simulink model "Electrical_System_2018b_obfs"  (R2019b)
settings: Solver=VariableStepAuto  StartTime=0.0  StopTime=5  RelTol=1e-3  AbsTol=1e-3  EnableMultiTasking=on
InitFcn:
  | Steady_State_Initialisation;
StopFcn:
  | %sscexplore(simlog);
  | %Logging
undefined symbols (not defined in the file): abrlhklxvp, aexgmhuedq, afmfmjnutg, afpphrjpnc, ahuxbyvruc, alarvljztt, amxnyqmnuw, aodrlwvqie, aolhmuplyq, aqpmguuqkg, auesgwirzl, aurophlnng, awamelrhru, ayfhvxflxn, azxkacuhqc, babszerikg, bawhdqanwq, bevoqecvei, bltjvqbchx, bmqsuewujl, bsmyqjfgnf, btvjbsmnve, bywgxqeadw, bziaduxaer, bzmcmdqocb, bzsvyvetat, ccsjnrbsih, cdvenygxwh, cedkrnslhx, cjheorclzs, cjrdshrtqx, ckhavyhcza, ckxewznhlz, cmrcgyiplk, conenicnws, cqkejbgjnn, csfnuwymhe, cunupkhwbh, cwzfvzuxxh, dcadmadufn, dcfponivnv, ddtrqjrhjn, dfhoxvkqas, dfrhtcwpne, dfvomcagjv, djijwylxea, dnmeqksrrm, dnzewbdkaa, dsqcykyxav, dtswwlttmm, ecumpidjtv, edegaywrct, ejjjsmnejc, eknqnehjdz, emvdetzouf, esxbqkbahr, etnkkbreiq, eunoiiiirw, ewewcuedir, fatkfxdhtc ... (+386)
libraries: fl_lib x802, ee_lib x362, fl_ps_legacy_lib x160, nesl_utility x85
(part 9 of 26)

== system Electrical_System_2018b_obfs/Redacted_1221/Redacted_7996/Redacted_1/Redacted_4377/Redacted_6082/Redacted_1335 ==
  Redacted_1591 : ee_lib/Semiconductors & Converters/Diode  ModelType=eepsypmlnm  Vf=vsdkpxkdvt V  Ron=hvipwyltcs Ohm  Goff=pncgtdpcky S  prmExp=ywnmgnebdg  I12=pijcksfllq A  V12=sokkewuwnq V  IS=lenjbmkbmu A  ec=usrydsfczj  I1=diflzejvue A  V1=ondqlqjixt V  RS=mmlszzuage Ohm  Tmeas=npymjxtxff degC  N_series=uwgycohtvj  N_parallel=vvktvyaksv  Rz=csndwjwvcs Ohm  BV=siuhniwsas V  C_param=mqmeyzacus  CJ=pspkjiflhw pF  CJ0=mkzhvuscrv pF  VJ=cxyxmemllb V  Mgrad=kwjdstgiqi  Vvec=rfkmbedwbl V  Cvec=tzcpccccyr pF  FC=tzhyramxnn  Q_param=jtaiadwcvb  iRM=teewqjimfa A  iF=dkuaowzmzk A  didt=wswqfekgti A/us  trr_factor=vgbmpjncqd  trr=qytitrwxvl ns  Qrr=jukjiwceed s*uA  TT=vfhkswzpii ns  tau=bcxefnpqla ns  T_param=knzoykoruc  IS_T2=wmrtfwgfyn A  I1_T2=wwatewxxmj A  V1_T2=vcmdipevcj V  Tmeas2=slejovgnym degC  EG_param=yrmdwgjpga  EG=obqdoxighd eV  XTI_param=hiiulsmtnp  XTI=fzvxbjgrlx  dBVdT=tcetjpxzuo V/K  Tdevice=jhymtvpuuv degC  i_specify=off  i_priority=None  i=lxkrvrufkt A  i_nominal_specify=off  i_nominal_unit=A  i_nominal_value=fptpkrapsh  v_specify=off  v_priority=None  v=hnwpggrdrb V  v_nominal_specify=off  v_nominal_unit=V  v_nominal_value=loyliznani  i_capacitor_specify=off  i_capacitor_priority=None  i_capacitor=qntetqcfew A  i_capacitor_nominal_specify=off  i_capacitor_nominal_unit=A  i_capacitor_nominal_value=bhetqfpmna  v_capacitor_specify=off  v_capacitor_priority=None  v_capacitor=qmuuchuxyz V  v_capacitor_nominal_specify=off  v_capacitor_nominal_unit=V  v_capacitor_nominal_value=vvvpkitexs  power_dissipated_specify=off  power_dissipated_priority=None  power_dissipated=kbjvtlpgfd W  power_dissipated_nominal_specify=off  power_dissipated_nominal_unit=W  power_dissipated_nominal_value=jvdnwocntn  thermal_network_parameterization=yoawbybtkl  Rth=uknyprueob K/W  Rth_Foster=quhjgsiudl K/W  thermal_mass_parameterization=atrvywscev  thermal_mass=gtmjoozywy J/K  thermal_mass_Foster=hdtqidrsds J/K  thermal_time_constant=adrtjfdoqm s  thermal_time_constant_Foster=lcosfsblai s  thermal_mass_initial_temperatures=kqftjagahg degC
      settings: SourceProductName=Simscape Electrical  InternalSimscapePortConfiguration="{\"Bottom\":[],\"Left\":[{\"id\":\"p\",\"label\":\"\",\"type\":\"foundation.electrical.electrical\"},{\"id\":\"H\",\"label\":\"H\",\"type\":\"foundation.thermal.thermal\"}],\"Right\":[{\"id\":\"n\",\"label\":\"\",\"type\":\"foundation.electrical.electrical\"}],\"Top\":[]}"
  Redacted_1669 : ee_lib/Passive/Thermal/Thermal Resistor  R=ejjjsmnejc K/W  T_specify=off  T_priority=None  T=mbytgkvqdk K  T_nominal_specify=off  T_nominal_unit=K  T_nominal_value=uvrqbhbcsu  Q_specify=off  Q_priority=None  Q=fryoumgfor W  Q_nominal_specify=off  Q_nominal_unit=W  Q_nominal_value=qudqfymccr
      settings: SourceProductName=Simscape Electrical  SourceProductBaseCode=PS  InternalSimscapePortConfiguration="{\"Bottom\":[],\"Left\":[{\"id\":\"A\",\"label\":\"A\",\"type\":\"foundation.thermal.thermal\"}],\"Right\":[{\"id\":\"B\",\"label\":\"B\",\"type\":\"foundation.thermal.thermal\"}],\"Top\":[]}"
  Redacted_4093 : fl_lib/Electrical/Electrical Elements/Switch  R_closed=bbadzxwyew Ohm  G_open=fzmtkxgwpd 1/Ohm  Threshold=dfvomcagjv  i_specify=off  i_priority=None  i=ohbeugqvip A  i_nominal_specify=off  i_nominal_unit=A  i_nominal_value=exxqjlbakz  v_specify=off  v_priority=None  v=rdiaxwucpj V  v_nominal_specify=off  v_nominal_unit=V  v_nominal_value=azkctcjsnz
      settings: SourceProductName=Simscape
  Redacted_5466 : ee_lib/Passive/Thermal/Thermal Resistor  R=wdtmondimm K/W  T_specify=off  T_priority=None  T=wrtafdzvbh K  T_nominal_specify=off  T_nominal_unit=K  T_nominal_value=fiihiabjan  Q_specify=off  Q_priority=None  Q=ypouestzei W  Q_nominal_specify=off  Q_nominal_unit=W  Q_nominal_value=mabqlhycjh
      settings: SourceProductName=Simscape Electrical  SourceProductBaseCode=PS  InternalSimscapePortConfiguration="{\"Bottom\":[],\"Left\":[{\"id\":\"A\",\"label\":\"A\",\"type\":\"foundation.thermal.thermal\"}],\"Right\":[{\"id\":\"B\",\"label\":\"B\",\"type\":\"foundation.thermal.thermal\"}],\"Top\":[]}"
  Redacted_7324 : fl_lib/Electrical/Electrical Elements/Switch  R_closed=omfvajnpfd Ohm  G_open=ipqnezpryn 1/Ohm  Threshold=mmcsavdyob  i_specify=off  i_priority=None  i=qwnjhvyruv A  i_nominal_specify=off  i_nominal_unit=A  i_nominal_value=zmauchnwye  v_specify=off  v_priority=None  v=ufnknxdamw V  v_nominal_specify=off  v_nominal_unit=V  v_nominal_value=edufhutzre
      settings: SourceProductName=Simscape
  Redacted_9050 : ee_lib/Passive/Thermal/Thermal Resistor  R=gnxjfqgycd K/W  T_specify=off  T_priority=None  T=dtswwlttmm K  T_nominal_specify=off  T_nominal_unit=K  T_nominal_value=iuxynuhpbk  Q_specify=off  Q_priority=None  Q=etqvxuddqu W  Q_nominal_specify=off  Q_nominal_unit=W  Q_nominal_value=jpdxcuslyz
      settings: SourceProductName=Simscape Electrical  SourceProductBaseCode=PS  InternalSimscapePortConfiguration="{\"Bottom\":[],\"Left\":[{\"id\":\"A\",\"label\":\"A\",\"type\":\"foundation.thermal.thermal\"}],\"Right\":[{\"id\":\"B\",\"label\":\"B\",\"type\":\"foundation.thermal.thermal\"}],\"Top\":[]}"
  Redacted_998 : ee_lib/Semiconductors & Converters/Diode  ModelType=jjfughauiv  Vf=eaqvjmxxyg V  Ron=canwxvkyyq Ohm  Goff=fylhafqfdf S  prmExp=dyvujabdmn  I12=kttaerjvea A  V12=kesibchmqe V  IS=cnmgoowrsx A  ec=wmgmtbxlpj  I1=kbcmpxrtrl A  V1=bxdgeigcbm V  RS=aqtkcecpuq Ohm  Tmeas=jagkxxxouu degC  N_series=eijeaxwsbs  N_parallel=gnezyptovg  Rz=ccfbjkqckh Ohm  BV=ibaqbmeitx V  C_param=qbielwnwyc  CJ=zriiuwgwxe pF  CJ0=dfescxdcew pF  VJ=cbwvhwuxfk V  Mgrad=imxnoqiriq  Vvec=scyvszjglj V  Cvec=fxqxkbblsd pF  FC=oefuhmbbrj  Q_param=azpytwrwfh  iRM=vffiognxml A  iF=obozmuzsag A  didt=gxjsoognzt A/us  trr_factor=ngilewgegt  trr=udeiywtgjk ns  Qrr=lseeyedphz s*uA  TT=rsgjgrebyr ns  tau=fnsxhspmvy ns  T_param=ompevgbwln  IS_T2=czoaxjmnms A  I1_T2=fomygjynsp A  V1_T2=axnvwvykbq V  Tmeas2=acusxjthih degC  EG_param=jvdcorncji  EG=cjbueeqdfy eV  XTI_param=ksyxmxcrgv  XTI=lqwkbkflhk  dBVdT=gzrvmvfdkg V/K  Tdevice=btlrowuowx degC  i_specify=off  i_priority=None  i=cbrwwtdksz A  i_nominal_specify=off  i_nominal_unit=A  i_nominal_value=tdaqsczgka  v_specify=off  v_priority=None  v=hzgsyifftd V  v_nominal_specify=off  v_nominal_unit=V  v_nominal_value=wwgtgaavtg  i_capacitor_specify=off  i_capacitor_priority=None  i_capacitor=ghdwybcfnr A  i_capacitor_nominal_specify=off  i_capacitor_nominal_unit=A  i_capacitor_nominal_value=patoccuvbb  v_capacitor_specify=off  v_capacitor_priority=None  v_capacitor=kipgljoorb V  v_capacitor_nominal_specify=off  v_capacitor_nominal_unit=V  v_capacitor_nominal_value=dyvrmzctdc  power_dissipated_specify=off  power_dissipated_priority=None  power_dissipated=ttfhebcktj W  power_dissipated_nominal_specify=off  power_dissipated_nominal_unit=W  power_dissipated_nominal_value=repcdnmkvu  thermal_network_parameterization=fmvbkiqdne  Rth=pazmfgafaa K/W  Rth_Foster=brspocefdd K/W  thermal_mass_parameterization=ykylewhfcq  thermal_mass=lrrjyxxvqd J/K  thermal_mass_Foster=vdbqyqwkrw J/K  thermal_time_constant=exusymqbix s  thermal_time_constant_Foster=asebieqyaj s  thermal_mass_initial_temperatures=hpkeovjooi degC
      settings: SourceProductName=Simscape Electrical  InternalSimscapePortConfiguration="{\"Bottom\":[],\"Left\":[{\"id\":\"p\",\"label\":\"\",\"type\":\"foundation.electrical.electrical\"},{\"id\":\"H\",\"label\":\"H\",\"type\":\"foundation.thermal.thermal\"}],\"Right\":[{\"id\":\"n\",\"label\":\"\",\"type\":\"foundation.electrical.electrical\"}],\"Top\":[]}"
  Redacted_3665 : PMIOPort  Side=Left
  Redacted_9500 : PMIOPort  Port=2  Side=Left
  Redacted_4916 : PMIOPort  Port=3  Side=Right
  Redacted_8865 : PMIOPort  Port=4  Side=Right
  Redacted_5813 : PMIOPort  Port=5  Side=Left
  Redacted_175 : PMIOPort  Port=6  Side=Right
  connections:
  Redacted_998/LConn2 -- Redacted_5466/LConn1
  Redacted_9050/RConn1 -- Redacted_5813/RConn1
  Redacted_8865/RConn1 -- Redacted_7324/RConn2
  Redacted_4093/RConn1 -- Redacted_7324/RConn1 -- Redacted_175/RConn1
  Redacted_1669/RConn1 -- Redacted_9050/LConn1 -- Redacted_5466/RConn1
  Redacted_3665/RConn1 -- Redacted_1591/RConn1
  Redacted_1591/LConn1 -- Redacted_4093/LConn1
  Redacted_4916/RConn1 -- Redacted_4093/RConn2
  Redacted_1591/LConn2 -- Redacted_1669/LConn1
  Redacted_998/RConn1 -- Redacted_7324/LConn1
  Redacted_998/LConn1 -- Redacted_9500/RConn1

== system Electrical_System_2018b_obfs/Redacted_1221/Redacted_7996/Redacted_1/Redacted_4377/Redacted_6082/Redacted_1337 ==
  Redacted_1292 : ee_lib/Passive/Thermal/Thermal Resistor  R=gfxbaoqbci K/W  T_specify=off  T_priority=None  T=rvwtgoykrz K  T_nominal_specify=off  T_nominal_unit=K  T_nominal_value=dmbpfjxefx  Q_specify=off  Q_priority=None  Q=ozjvrxmttl W  Q_nominal_specify=off  Q_nominal_unit=W  Q_nominal_value=utwlydmrkv
      settings: SourceProductName=Simscape Electrical  SourceProductBaseCode=PS  InternalSimscapePortConfiguration="{\"Bottom\":[],\"Left\":[{\"id\":\"A\",\"label\":\"A\",\"type\":\"foundation.thermal.thermal\"}],\"Right\":[{\"id\":\"B\",\"label\":\"B\",\"type\":\"foundation.thermal.thermal\"}],\"Top\":[]}"
  Redacted_2743 : fl_lib/Electrical/Electrical Elements/Switch  R_closed=fsyfpyiukg Ohm  G_open=tvcalsacmg 1/Ohm  Threshold=ttjzchmxti  i_specify=off  i_priority=None  i=alduyvsbin A  i_nominal_specify=off  i_nominal_unit=A  i_nominal_value=loyuiwztoz  v_specify=off  v_priority=None  v=yjwvqchbme V  v_nominal_specify=off  v_nominal_unit=V  v_nominal_value=gjoornamne
      settings: SourceProductName=Simscape
  Redacted_3949 : ee_lib/Passive/Thermal/Thermal Resistor  R=mlcqaguecq K/W  T_specify=off  T_priority=None  T=hfikrglmxq K  T_nominal_specify=off  T_nominal_unit=K  T_nominal_value=dqcyvveaih  Q_specify=off  Q_priority=None  Q=qlchfeptuj W  Q_nominal_specify=off  Q_nominal_unit=W  Q_nominal_value=wfdtozcpan
      settings: SourceProductName=Simscape Electrical  SourceProductBaseCode=PS  InternalSimscapePortConfiguration="{\"Bottom\":[],\"Left\":[{\"id\":\"A\",\"label\":\"A\",\"type\":\"foundation.thermal.thermal\"}],\"Right\":[{\"id\":\"B\",\"label\":\"B\",\"type\":\"foundation.thermal.thermal\"}],\"Top\":[]}"
  Redacted_4700 : ee_lib/Passive/Thermal/Thermal Resistor  R=gvbddagohg K/W  T_specify=off  T_priority=None  T=qxaoehcsep K  T_nominal_specify=off  T_nominal_unit=K  T_nominal_value=nuvljcivmd  Q_specify=off  Q_priority=None  Q=cuqzitalwz W  Q_nominal_specify=off  Q_nominal_unit=W  Q_nominal_value=fpqwunqvoe
      settings: SourceProductName=Simscape Electrical  SourceProductBaseCode=PS  InternalSimscapePortConfiguration="{\"Bottom\":[],\"Left\":[{\"id\":\"A\",\"label\":\"A\",\"type\":\"foundation.thermal.thermal\"}],\"Right\":[{\"id\":\"B\",\"label\":\"B\",\"type\":\"foundation.thermal.thermal\"}],\"Top\":[]}"
  Redacted_6636 : fl_lib/Electrical/Electrical Elements/Switch  R_closed=cxbeobdwcz Ohm  G_open=vivqqcjshk 1/Ohm  Threshold=ihvrcphyhk  i_specify=off  i_priority=None  i=tlqvhosmyx A  i_nominal_specify=off  i_nominal_unit=A  i_nominal_value=zlqewbizhg  v_specify=off  v_priority=None  v=bylehoytgr V  v_nominal_specify=off  v_nominal_unit=V  v_nominal_value=nrfabisoae
      settings: SourceProductName=Simscape
  Redacted_7671 : ee_lib/Semiconductors & Converters/Diode  ModelType=olgpyqkyap  Vf=yiidzvusor V  Ron=onikhigqex Ohm  Goff=zwvbfgfjia S  prmExp=mbejlzmzoi  I12=iqvhxxtdcy A  V12=plenerjsyz V  IS=seajxixdni A  ec=smzaoqkpfi  I1=srlrouujzp A  V1=pbinkrtesx V  RS=maerkwpvvt Ohm  Tmeas=boxaemfztm degC  N_series=zwoiykegtu  N_parallel=jpsnlhanqe  Rz=rbegpmpdpq Ohm  BV=xqcgehksui V  C_param=smmkeyjtrn  CJ=mxoawofixc pF  CJ0=ucwkumcrgx pF  VJ=flpomdjhqn V  Mgrad=pogzifmwhx  Vvec=lvysrprkky V  Cvec=ofowmtrtdp pF  FC=xzrncupysx  Q_param=dpijdlsbtg  iRM=imlwlhdaoz A  iF=zahcqmmmsp A  didt=srqymkpvtu A/us  trr_factor=qutyflkerp  trr=alnpfsdzft ns  Qrr=pnoodsbkqz s*uA  TT=qzjfylnffu ns  tau=fiwiuyhrdw ns  T_param=wjqxjtpsrv  IS_T2=gnlmqposwz A  I1_T2=hhxkfrkipw A  V1_T2=otwkxldrvh V  Tmeas2=pqzzkcslrw degC  EG_param=rgdwepjzgz  EG=towtzjxupc eV  XTI_param=wnrxgiphjy  XTI=ifqnzmcann  dBVdT=izcgyclarw V/K  Tdevice=kuguckrfas degC  i_specify=off  i_priority=None  i=qwraxdsfza A  i_nominal_specify=off  i_nominal_unit=A  i_nominal_value=jrebnsmptq  v_specify=off  v_priority=None  v=faivdficoh V  v_nominal_specify=off  v_nominal_unit=V  v_nominal_value=bfbyoqyboc  i_capacitor_specify=off  i_capacitor_priority=None  i_capacitor=jrptblagdq A  i_capacitor_nominal_specify=off  i_capacitor_nominal_unit=A  i_capacitor_nominal_value=nibfyfosby  v_capacitor_specify=off  v_capacitor_priority=None  v_capacitor=whspnfsgdn V  v_capacitor_nominal_specify=off  v_capacitor_nominal_unit=V  v_capacitor_nominal_value=edempxzddr  power_dissipated_specify=off  power_dissipated_priority=None  power_dissipated=peqvvccveb W  power_dissipated_nominal_specify=off  power_dissipated_nominal_unit=W  power_dissipated_nominal_value=fvdlfslssq  thermal_network_parameterization=svzrqymosw  Rth=pzdrjrnlgr K/W  Rth_Foster=acztezytnk K/W  thermal_mass_parameterization=rgscyvsrgf  thermal_mass=kygdzlscru J/K  thermal_mass_Foster=dvwwklbogc J/K  thermal_time_constant=ykfmdcuqty s  thermal_time_constant_Foster=wgtknjdmmg s  thermal_mass_initial_temperatures=gjuzcynxks degC
      settings: SourceProductName=Simscape Electrical  InternalSimscapePortConfiguration="{\"Bottom\":[],\"Left\":[{\"id\":\"p\",\"label\":\"\",\"type\":\"foundation.electrical.electrical\"},{\"id\":\"H\",\"label\":\"H\",\"type\":\"foundation.thermal.thermal\"}],\"Right\":[{\"id\":\"n\",\"label\":\"\",\"type\":\"foundation.electrical.electrical\"}],\"Top\":[]}"
  Redacted_7804 : ee_lib/Semiconductors & Converters/Diode  ModelType=semwhebdsx  Vf=wlzsjodvxe V  Ron=kjejwwsved Ohm  Goff=idmqtjqxyt S  prmExp=ybznmgfoim  I12=ypbwuazhvu A  V12=kqbjrekczm V  IS=hvghirmuer A  ec=szvhwtedho  I1=dgebikxuyu A  V1=ekmofvolqe V  RS=jkmhfachtm Ohm  Tmeas=ahwyvfcpsr degC  N_series=atodrtceph  N_parallel=fkaurojkbb  Rz=egfgmfcnxn Ohm  BV=nluxtwjaqz V  C_param=qwanuoxlyf  CJ=ezbprdeztn pF  CJ0=peskbsrzop pF  VJ=vquvaidumd V  Mgrad=dfrmgpetae  Vvec=gunyxlsjla V  Cvec=nljyfkzkue pF  FC=itkqjjkjyc  Q_param=jgelcbblhx  iRM=jgdtjqhets A  iF=owsoaymscw A  didt=qmpgbmxkte A/us  trr_factor=hklhqkgxog  trr=veyznjjddh ns  Qrr=ejjniorttw s*uA  TT=suevkibuvy ns  tau=mawzmcgeyp ns  T_param=vqrqwbsxyj  IS_T2=ssgvnzergm A  I1_T2=kvtrmiebrl A  V1_T2=wfzbyspvvb V  Tmeas2=oidirsmqgk degC  EG_param=zfeizsafro  EG=pynrradmvc eV  XTI_param=chffuchcuy  XTI=acqdodawvu  dBVdT=ocrbmtpnpr V/K  Tdevice=zuabybkowd degC  i_specify=off  i_priority=None  i=bcjxinvzmi A  i_nominal_specify=off  i_nominal_unit=A  i_nominal_value=ackfofeggx  v_specify=off  v_priority=None  v=nodroimedg V  v_nominal_specify=off  v_nominal_unit=V  v_nominal_value=nhpkywzxmk  i_capacitor_specify=off  i_capacitor_priority=None  i_capacitor=gbqfpnudcs A  i_capacitor_nominal_specify=off  i_capacitor_nominal_unit=A  i_capacitor_nominal_value=jfrtogbkdj  v_capacitor_specify=off  v_capacitor_priority=None  v_capacitor=kykdbedtbj V  v_capacitor_nominal_specify=off  v_capacitor_nominal_unit=V  v_capacitor_nominal_value=bwzkdbziru  power_dissipated_specify=off  power_dissipated_priority=None  power_dissipated=crijfdzbch W  power_dissipated_nominal_specify=off  power_dissipated_nominal_unit=W  power_dissipated_nominal_value=gueeagjtzs  thermal_network_parameterization=nshhtosrtp  Rth=ymvhergmsa K/W  Rth_Foster=loktjbqqnk K/W  thermal_mass_parameterization=nxtgvvflim  thermal_mass=ipqsjmpyeh J/K  thermal_mass_Foster=pnnymgjcyt J/K  thermal_time_constant=fqlitfupll s  thermal_time_constant_Foster=ouoyijytio s  thermal_mass_initial_temperatures=hosplxrwnn degC
      settings: SourceProductName=Simscape Electrical  InternalSimscapePortConfiguration="{\"Bottom\":[],\"Left\":[{\"id\":\"p\",\"label\":\"\",\"type\":\"foundation.electrical.electrical\"},{\"id\":\"H\",\"label\":\"H\",\"type\":\"foundation.thermal.thermal\"}],\"Right\":[{\"id\":\"n\",\"label\":\"\",\"type\":\"foundation.electrical.electrical\"}],\"Top\":[]}"
  Redacted_9723 : PMIOPort  Side=Left
  Redacted_1721 : PMIOPort  Port=2  Side=Left
  Redacted_9002 : PMIOPort  Port=3  Side=Right
  Redacted_1469 : PMIOPort  Port=4  Side=Right
  Redacted_6509 : PMIOPort  Port=5  Side=Left
  Redacted_1134 : PMIOPort  Port=6  Side=Right
  connections:
  Redacted_7671/LConn2 -- Redacted_3949/LConn1
  Redacted_4700/RConn1 -- Redacted_6509/RConn1
  Redacted_1469/RConn1 -- Redacted_6636/RConn2
  Redacted_2743/RConn1 -- Redacted_6636/RConn1 -- Redacted_1134/RConn1
  Redacted_1292/RConn1 -- Redacted_4700/LConn1 -- Redacted_3949/RConn1
  Redacted_9723/RConn1 -- Redacted_7804/RConn1
  Redacted_7804/LConn1 -- Redacted_2743/LConn1
  Redacted_9002/RConn1 -- Redacted_2743/RConn2
  Redacted_7804/LConn2 -- Redacted_1292/LConn1
  Redacted_7671/RConn1 -- Redacted_6636/LConn1
  Redacted_7671/LConn1 -- Redacted_1721/RConn1

== system Electrical_System_2018b_obfs/Redacted_1221/Redacted_7996/Redacted_1/Redacted_4377/Redacted_6082/Redacted_144 ==
  Neutral_Negative : Subsystem  VariantControl=Variant1
  Positive_Neutral : Subsystem  VariantControl=Variant3
  Redacted_9503 : Subsystem  VariantControl=Variant2
  Redacted_3879 : PMIOPort  Side=Left
  Redacted_3368 : PMIOPort  Port=2  Side=Left
  Redacted_9451 : PMIOPort  Port=3  Side=Left
  Redacted_8432 : PMIOPort  Port=4  Side=Right
  Redacted_6806 : PMIOPort  Port=5  Side=Right

== system Electrical_System_2018b_obfs/Redacted_1221/Redacted_7996/Redacted_1/Redacted_4377/Redacted_6082/Redacted_1502 ==
  Redacted_179 : fl_lib/Electrical/Electrical Elements/Switch  R_closed=tpfczkzopb Ohm  G_open=guejjlojqy 1/Ohm  Threshold=qftxyxgxji  i_specify=off  i_priority=None  i=fngbtljzex A  i_nominal_specify=off  i_nominal_unit=A  i_nominal_value=pjpooffzff  v_specify=off  v_priority=None  v=bhcpirmmxz V  v_nominal_specify=off  v_nominal_unit=V  v_nominal_value=jucxroftek
      settings: SourceProductName=Simscape
  Redacted_1815 : ee_lib/Semiconductors & Converters/Diode  ModelType=dqnklwqfci  Vf=xjiqjpnnfi V  Ron=irekdgqkjv Ohm  Goff=iqhtpofome S  prmExp=knojfylagq  I12=bqxijupuhm A  V12=vzuzujtkpl V  IS=ydgywotbys A  ec=ayrfemqefn  I1=delsjshmli A  V1=dnxxzmtubb V  RS=wmjpjwroih Ohm  Tmeas=qmtcdggbzc degC  N_series=hklouwtkux  N_parallel=jrdkdmsmgo  Rz=tovmqbbrol Ohm  BV=avdgidxjam V  C_param=glqkxeqcta  CJ=chsawhndir pF  CJ0=ayexifqzkz pF  VJ=zqcsdkhphs V  Mgrad=fkespxnvnl  Vvec=dqwhbiesyc V  Cvec=niiqpqslou pF  FC=cwbzovuqpz  Q_param=ylelzifboz  iRM=omgsmfewsp A  iF=ichmjhkctu A  didt=orrasyxhrt A/us  trr_factor=zdlyciflht  trr=twfpakhxfd ns  Qrr=ipntneuszo s*uA  TT=mwhbnzgoop ns  tau=pfrrcdfsln ns  T_param=ytujlpikwb  IS_T2=jerhvoexxa A  I1_T2=jvyzqlfhuc A  V1_T2=zarbmnbtma V  Tmeas2=vwndrphzjd degC  EG_param=pcxlgqdkwd  EG=vtwlzbuxst eV  XTI_param=jcpfqvyxtb  XTI=phmgnxxjxe  dBVdT=orxkvsgthq V/K  Tdevice=oqbwtmobso degC  i_specify=off  i_priority=None  i=yajbkzqnsh A  i_nominal_specify=off  i_nominal_unit=A  i_nominal_value=iwrztftqvf  v_specify=off  v_priority=None  v=ewtusmxpho V  v_nominal_specify=off  v_nominal_unit=V  v_nominal_value=syahoyjouu  i_capacitor_specify=off  i_capacitor_priority=None  i_capacitor=vxlszklfgf A  i_capacitor_nominal_specify=off  i_capacitor_nominal_unit=A  i_capacitor_nominal_value=duzmsfhmfv  v_capacitor_specify=off  v_capacitor_priority=None  v_capacitor=grvkfvfijd V  v_capacitor_nominal_specify=off  v_capacitor_nominal_unit=V  v_capacitor_nominal_value=zqixbhndtz  power_dissipated_specify=off  power_dissipated_priority=None  power_dissipated=bveezoguoz W  power_dissipated_nominal_specify=off  power_dissipated_nominal_unit=W  power_dissipated_nominal_value=wuvllpdufa  thermal_network_parameterization=rsoaylhfgu  Rth=owtikceqjs K/W  Rth_Foster=lmkblyjvxa K/W  thermal_mass_parameterization=edoczwbxzz  thermal_mass=ujhryaplvc J/K  thermal_mass_Foster=jnfsbuuslg J/K  thermal_time_constant=psujdozuva s  thermal_time_constant_Foster=kopgklxeqj s  thermal_mass_initial_temperatures=hdbyfhhyky degC
      settings: SourceProductName=Simscape Electrical  InternalSimscapePortConfiguration="{\"Bottom\":[],\"Left\":[{\"id\":\"p\",\"label\":\"\",\"type\":\"foundation.electrical.electrical\"},{\"id\":\"H\",\"label\":\"H\",\"type\":\"foundation.thermal.thermal\"}],\"Right\":[{\"id\":\"n\",\"label\":\"\",\"type\":\"foundation.electrical.electrical\"}],\"Top\":[]}"
  Redacted_309 : ee_lib/Passive/Thermal/Thermal Resistor  R=rlqpvmzzkw K/W  T_specify=off  T_priority=None  T=fayvhqopgz K  T_nominal_specify=off  T_nominal_unit=K  T_nominal_value=usakfhvqjr  Q_specify=off  Q_priority=None  Q=fradxufojf W  Q_nominal_specify=off  Q_nominal_unit=W  Q_nominal_value=vqlkwzshfu
      settings: SourceProductName=Simscape Electrical  SourceProductBaseCode=PS  InternalSimscapePortConfiguration="{\"Bottom\":[],\"Left\":[{\"id\":\"A\",\"label\":\"A\",\"type\":\"foundation.thermal.thermal\"}],\"Right\":[{\"id\":\"B\",\"label\":\"B\",\"type\":\"foundation.thermal.thermal\"}],\"Top\":[]}"
  Redacted_5427 : ee_lib/Semiconductors & Converters/Diode  ModelType=pvrilldlsl  Vf=exnaqxwczp V  Ron=byxhoupfbl Ohm  Goff=cclixdjcai S  prmExp=zgdvwqebkp  I12=aaaajndugd A  V12=zehnejyycd V  IS=bhumfyvqsp A  ec=qksjfmhjtn  I1=dzbxvwsdwy A  V1=qmphnapbom V  RS=ctsixmdfmz Ohm  Tmeas=voedtwdeem degC  N_series=zgsqwpgvsr  N_parallel=uokulxwqht  Rz=wfrfbwnojp Ohm  BV=qeyzssoejo V  C_param=svrqcrwtfc  CJ=dnwihzlyai pF  CJ0=qnrhvsekkn pF  VJ=qwvipkfmhu V  Mgrad=aiprwlrmva  Vvec=virrpuurya V  Cvec=inrcnfmckm pF  FC=vrvicjveyg  Q_param=uayuuepkqf  iRM=ktwoixrfbu A  iF=agmjhjxbxi A  didt=wopacoyifj A/us  trr_factor=mctfeqcgzf  trr=mcokfacpzx ns  Qrr=rvqtwqbvse s*uA  TT=wzilqodkkq ns  tau=ovarvjbymx ns  T_param=eagmvacwck  IS_T2=gceloirlpi A  I1_T2=cuojdhyufm A  V1_T2=ddoadsxlun V  Tmeas2=owwfcnzgyt degC  EG_param=htmtzkabpk  EG=znuuglnooo eV  XTI_param=rlgyybapxj  XTI=chmfxclcvd  dBVdT=mndckszxsr V/K  Tdevice=earqsgdndu degC  i_specify=off  i_priority=None  i=paejymtbgc A  i_nominal_specify=off  i_nominal_unit=A  i_nominal_value=ghormagyrn  v_specify=off  v_priority=None  v=mlxeomuyaz V  v_nominal_specify=off  v_nominal_unit=V  v_nominal_value=uzogtcjxmk  i_capacitor_specify=off  i_capacitor_priority=None  i_capacitor=reqkofmrwn A  i_capacitor_nominal_specify=off  i_capacitor_nominal_unit=A  i_capacitor_nominal_value=ofzxyeyrlg  v_capacitor_specify=off  v_capacitor_priority=None  v_capacitor=genvugjiwl V  v_capacitor_nominal_specify=off  v_capacitor_nominal_unit=V  v_capacitor_nominal_value=luaqihueqh  power_dissipated_specify=off  power_dissipated_priority=None  power_dissipated=xzkkuqjorb W  power_dissipated_nominal_specify=off  power_dissipated_nominal_unit=W  power_dissipated_nominal_value=gfhgakjqou  thermal_network_parameterization=kxvmefjoct  Rth=umlvscqlhx K/W  Rth_Foster=nlxizvbfxv K/W  thermal_mass_parameterization=yrswehzqhv  thermal_mass=uqwhhdrfmw J/K  thermal_mass_Foster=hjdthzjyej J/K  thermal_time_constant=fafhujuybb s  thermal_time_constant_Foster=rempkthvvv s  thermal_mass_initial_temperatures=zrogtrgfqe degC
      settings: SourceProductName=Simscape Electrical  InternalSimscapePortConfiguration="{\"Bottom\":[],\"Left\":[{\"id\":\"p\",\"label\":\"\",\"type\":\"foundation.electrical.electrical\"},{\"id\":\"H\",\"label\":\"H\",\"type\":\"foundation.thermal.thermal\"}],\"Right\":[{\"id\":\"n\",\"label\":\"\",\"type\":\"foundation.electrical.electrical\"}],\"Top\":[]}"
  Redacted_8072 : fl_lib/Electrical/Electrical Elements/Switch  R_closed=gnicoyhwdb Ohm  G_open=bwtrzzqkxe 1/Ohm  Threshold=btvjbsmnve  i_specify=off  i_priority=None  i=ffgvusnnup A  i_nominal_specify=off  i_nominal_unit=A  i_nominal_value=olaaofnvmv  v_specify=off  v_priority=None  v=hazqywjesu V  v_nominal_specify=off  v_nominal_unit=V  v_nominal_value=cujoeegpfv
      settings: SourceProductName=Simscape
  Redacted_8744 : ee_lib/Passive/Thermal/Thermal Resistor  R=qiiyhvuybo K/W  T_specify=off  T_priority=None  T=bmqsuewujl K  T_nominal_specify=off  T_nominal_unit=K  T_nominal_value=vyegnflrcg  Q_specify=off  Q_priority=None  Q=ozzgwrnnpp W  Q_nominal_specify=off  Q_nominal_unit=W  Q_nominal_value=zifsigreky
      settings: SourceProductName=Simscape Electrical  SourceProductBaseCode=PS  InternalSimscapePortConfiguration="{\"Bottom\":[],\"Left\":[{\"id\":\"A\",\"label\":\"A\",\"type\":\"foundation.thermal.thermal\"}],\"Right\":[{\"id\":\"B\",\"label\":\"B\",\"type\":\"foundation.thermal.thermal\"}],\"Top\":[]}"
  Redacted_9404 : ee_lib/Passive/Thermal/Thermal Resistor  R=vbnoxlgcgw K/W  T_specify=off  T_priority=None  T=umlukkevvv K  T_nominal_specify=off  T_nominal_unit=K  T_nominal_value=tnumztnkxu  Q_specify=off  Q_priority=None  Q=kisoetcdki W  Q_nominal_specify=off  Q_nominal_unit=W  Q_nominal_value=kojngerfgf
      settings: SourceProductName=Simscape Electrical  SourceProductBaseCode=PS  InternalSimscapePortConfiguration="{\"Bottom\":[],\"Left\":[{\"id\":\"A\",\"label\":\"A\",\"type\":\"foundation.thermal.thermal\"}],\"Right\":[{\"id\":\"B\",\"label\":\"B\",\"type\":\"foundation.thermal.thermal\"}],\"Top\":[]}"
  Redacted_6664 : PMIOPort  Side=Left
  Redacted_9877 : PMIOPort  Port=2  Side=Left
  Redacted_7484 : PMIOPort  Port=3  Side=Right
  Redacted_239 : PMIOPort  Port=4  Side=Right
  Redacted_1077 : PMIOPort  Port=5  Side=Left
  Redacted_1415 : PMIOPort  Port=6  Side=Right
  connections:
  Redacted_1815/LConn2 -- Redacted_309/LConn1
  Redacted_8744/RConn1 -- Redacted_1077/RConn1
  Redacted_239/RConn1 -- Redacted_179/RConn2
  Redacted_8072/RConn1 -- Redacted_179/RConn1 -- Redacted_1415/RConn1
  Redacted_9404/RConn1 -- Redacted_8744/LConn1 -- Redacted_309/RConn1
  Redacted_6664/RConn1 -- Redacted_5427/RConn1
  Redacted_5427/LConn1 -- Redacted_8072/LConn1
  Redacted_7484/RConn1 -- Redacted_8072/RConn2
  Redacted_5427/LConn2 -- Redacted_9404/LConn1
  Redacted_1815/RConn1 -- Redacted_179/LConn1
  Redacted_1815/LConn1 -- Redacted_9877/RConn1

== system Electrical_System_2018b_obfs/Redacted_1221/Redacted_7996/Redacted_1/Redacted_4377/Redacted_6082/Redacted_1544 ==
  Neutral_Negative : Subsystem  VariantControl=Variant1
  Positive_Neutral : Subsystem  VariantControl=Variant3
  Redacted_4672 : Subsystem  VariantControl=Variant2
  Redacted_697 : PMIOPort  Side=Left
  Redacted_9789 : PMIOPort  Port=2  Side=Left
  Redacted_5820 : PMIOPort  Port=3  Side=Left
  Redacted_1167 : PMIOPort  Port=4  Side=Right
  Redacted_9408 : PMIOPort  Port=5  Side=Right

== system Electrical_System_2018b_obfs/Redacted_1221/Redacted_7996/Redacted_1/Redacted_4377/Redacted_6082/Redacted_1658 ==
  Redacted_1005 : fl_lib/Electrical/Electrical Elements/Switch  R_closed=ejlyeridsw Ohm  G_open=efsydslasd 1/Ohm  Threshold=qludltxvzj  i_specify=off  i_priority=None  i=qtqqggocjg A  i_nominal_specify=off  i_nominal_unit=A  i_nominal_value=irfgdwsyws  v_specify=off  v_priority=None  v=nrsfaplzum V  v_nominal_specify=off  v_nominal_unit=V  v_nominal_value=ffnnoojtnr
      settings: SourceProductName=Simscape
  Redacted_1354 : ee_lib/Passive/Thermal/Thermal Resistor  R=qdgpqkdjpo K/W  T_specify=off  T_priority=None  T=mtinxqvpod K  T_nominal_specify=off  T_nominal_unit=K  T_nominal_value=nyetipzdbd  Q_specify=off  Q_priority=None  Q=zeibppilau W  Q_nominal_specify=off  Q_nominal_unit=W  Q_nominal_value=ovthkmdajp
      settings: SourceProductName=Simscape Electrical  SourceProductBaseCode=PS  InternalSimscapePortConfiguration="{\"Bottom\":[],\"Left\":[{\"id\":\"A\",\"label\":\"A\",\"type\":\"foundation.thermal.thermal\"}],\"Right\":[{\"id\":\"B\",\"label\":\"B\",\"type\":\"foundation.thermal.thermal\"}],\"Top\":[]}"
  Redacted_3286 : ee_lib/Semiconductors & Converters/Diode  ModelType=qyiuharngl  Vf=uavesysmzd V  Ron=izxucsnofw Ohm  Goff=hxvsqjqvfr S  prmExp=jwlbdrgdyn  I12=fhtaelyvur A  V12=pntclgauty V  IS=xlgdpvdion A  ec=lsuwwyvoaz  I1=xioaihhcoe A  V1=prlupfwjwk V  RS=grfujeuioo Ohm  Tmeas=mmahtgxtlp degC  N_series=bdqkkbdoww  N_parallel=bdgudnfeam  Rz=vsyxoldpzj Ohm  BV=rczxpthhgf V  C_param=tlcavagjol  CJ=ssqnkrbywq pF  CJ0=wrromkkilg pF  VJ=faazhshxub V  Mgrad=ldrovslsoh  Vvec=vtbaecghrb V  Cvec=rijvdbsbjz pF  FC=ouvrtbvulr  Q_param=rrrehddltc  iRM=fyquguupcf A  iF=ikkfryheqp A  didt=scbuuymmti A/us  trr_factor=vwdzzjgtdl  trr=zktlrrknks ns  Qrr=utuviybabn s*uA  TT=jcgggencbc ns  tau=ssflxvsiut ns  T_param=nblvkicsaj  IS_T2=hpuqfgybtl A  I1_T2=atejcpbsmg A  V1_T2=txapzmzmbr V  Tmeas2=hogrcmodsn degC  EG_param=fwyzdxmfgf  EG=zfrilvllus eV  XTI_param=gxndnzccej  XTI=zngcdbbpek  dBVdT=ultmrnqodj V/K  Tdevice=cvuddcjgoa degC  i_specify=off  i_priority=None  i=xckzxtcuri A  i_nominal_specify=off  i_nominal_unit=A  i_nominal_value=mfjascwvwx  v_specify=off  v_priority=None  v=oytsestkkt V  v_nominal_specify=off  v_nominal_unit=V  v_nominal_value=rbtpehkrox  i_capacitor_specify=off  i_capacitor_priority=None  i_capacitor=lydrbpwfwm A  i_capacitor_nominal_specify=off  i_capacitor_nominal_unit=A  i_capacitor_nominal_value=gsonjyrsiu  v_capacitor_specify=off  v_capacitor_priority=None  v_capacitor=tlqtmxeebh V  v_capacitor_nominal_specify=off  v_capacitor_nominal_unit=V  v_capacitor_nominal_value=ixflknqnnv  power_dissipated_specify=off  power_dissipated_priority=None  power_dissipated=vhmskoronr W  power_dissipated_nominal_specify=off  power_dissipated_nominal_unit=W  power_dissipated_nominal_value=rqgtxqlwdp  thermal_network_parameterization=xkaopcnmoj  Rth=skumtgliel K/W  Rth_Foster=widqwnvljq K/W  thermal_mass_parameterization=ihdtigkqdr  thermal_mass=fxsrzmeque J/K  thermal_mass_Foster=cbmthsfafj J/K  thermal_time_constant=pmaqruvvqr s  thermal_time_constant_Foster=pxvwqyklyc s  thermal_mass_initial_temperatures=qerohrajht degC
      settings: SourceProductName=Simscape Electrical  InternalSimscapePortConfiguration="{\"Bottom\":[],\"Left\":[{\"id\":\"p\",\"label\":\"\",\"type\":\"foundation.electrical.electrical\"},{\"id\":\"H\",\"label\":\"H\",\"type\":\"foundation.thermal.thermal\"}],\"Right\":[{\"id\":\"n\",\"label\":\"\",\"type\":\"foundation.electrical.electrical\"}],\"Top\":[]}"
  Redacted_3861 : ee_lib/Semiconductors & Converters/Diode  ModelType=fxgsrmkiul  Vf=nwkiuphnod V  Ron=ytonkdenqd Ohm  Goff=vvxokjkhhi S  prmExp=rjijseurnu  I12=plnpdpppsb A  V12=clscpnwkyn V  IS=fgyrvtcpjw A  ec=myarsmgyax  I1=zaiuznwqub A  V1=urqjkvkqaz V  RS=atpbcqwqrk Ohm  Tmeas=avxaumhyvi degC  N_series=bdgfkyrlsu  N_parallel=cgmwatvtyk  Rz=jwremjkbfv Ohm  BV=kmqlppxuzg V  C_param=vvtbjwiqjw  CJ=dvukuyjagk pF  CJ0=ajovvjufex pF  VJ=lqxioxyjxp V  Mgrad=ugprrqpcng  Vvec=aycruakske V  Cvec=grqlqlzqyb pF  FC=xafzerxcin  Q_param=vnlbkyokpw  iRM=myuopxdhnp A  iF=wopzcdppvb A  didt=yoejpqomll A/us  trr_factor=vnzcsazbfp  trr=flnrjlmhdl ns  Qrr=abhmmrvgxl s*uA  TT=gfztyjvgqq ns  tau=oustnvpcaz ns  T_param=aznyhdnxgk  IS_T2=boxomshjpr A  I1_T2=imlgomczsp A  V1_T2=bhyftvbhbd V  Tmeas2=bhksuazwhb degC  EG_param=asaybnfknm  EG=gsrzwalape eV  XTI_param=duwkdllyki  XTI=aszcjfwkon  dBVdT=xhavbsykud V/K  Tdevice=nfydvwwomt degC  i_specify=off  i_priority=None  i=hibpeusmqj A  i_nominal_specify=off  i_nominal_unit=A  i_nominal_value=dgpnvsgdwn  v_specify=off  v_priority=None  v=xzghpqhkll V  v_nominal_specify=off  v_nominal_unit=V  v_nominal_value=aqwbnuvuma  i_capacitor_specify=off  i_capacitor_priority=None  i_capacitor=dbdawzejgx A  i_capacitor_nominal_specify=off  i_capacitor_nominal_unit=A  i_capacitor_nominal_value=skfhqqsyjv  v_capacitor_specify=off  v_capacitor_priority=None  v_capacitor=kngohrnxjb V  v_capacitor_nominal_specify=off  v_capacitor_nominal_unit=V  v_capacitor_nominal_value=knpvixzgdi  power_dissipated_specify=off  power_dissipated_priority=None  power_dissipated=zhfsmmbryx W  power_dissipated_nominal_specify=off  power_dissipated_nominal_unit=W  power_dissipated_nominal_value=oxbqwsyfdo  thermal_network_parameterization=gluxlhswsh  Rth=wkzzkloygz K/W  Rth_Foster=lchzecrkjz K/W  thermal_mass_parameterization=gwvmgktbjo  thermal_mass=rmhlykpfbd J/K  thermal_mass_Foster=ahdrbmndbt J/K  thermal_time_constant=geccsojpnx s  thermal_time_constant_Foster=oeduphnpru s  thermal_mass_initial_temperatures=wnupirfodr degC
      settings: SourceProductName=Simscape Electrical  InternalSimscapePortConfiguration="{\"Bottom\":[],\"Left\":[{\"id\":\"p\",\"label\":\"\",\"type\":\"foundation.electrical.electrical\"},{\"id\":\"H\",\"label\":\"H\",\"type\":\"foundation.thermal.thermal\"}],\"Right\":[{\"id\":\"n\",\"label\":\"\",\"type\":\"foundation.electrical.electrical\"}],\"Top\":[]}"
  Redacted_5977 : fl_lib/Electrical/Electrical Elements/Switch  R_closed=cjwmmdrupk Ohm  G_open=qstxdugiyk 1/Ohm  Threshold=kztcpnpmvs  i_specify=off  i_priority=None  i=lmxbtdndwg A  i_nominal_specify=off  i_nominal_unit=A  i_nominal_value=qyeufjvfiw  v_specify=off  v_priority=None  v=gastazzonl V  v_nominal_specify=off  v_nominal_unit=V  v_nominal_value=mjiwwishzy
      settings: SourceProductName=Simscape
  Redacted_6041 : ee_lib/Passive/Thermal/Thermal Resistor  R=xbcnqysxek K/W  T_specify=off  T_priority=None  T=bzsvyvetat K  T_nominal_specify=off  T_nominal_unit=K  T_nominal_value=ewqiuajrkb  Q_specify=off  Q_priority=None  Q=jhzrvwpmgk W  Q_nominal_specify=off  Q_nominal_unit=W  Q_nominal_value=tohlmuixqc
      settings: SourceProductName=Simscape Electrical  SourceProductBaseCode=PS  InternalSimscapePortConfiguration="{\"Bottom\":[],\"Left\":[{\"id\":\"A\",\"label\":\"A\",\"type\":\"foundation.thermal.thermal\"}],\"Right\":[{\"id\":\"B\",\"label\":\"B\",\"type\":\"foundation.thermal.thermal\"}],\"Top\":[]}"
  Redacted_7612 : ee_lib/Passive/Thermal/Thermal Resistor  R=ogtgsqkykv K/W  T_specify=off  T_priority=None  T=welbpoxbdd K  T_nominal_specify=off  T_nominal_unit=K  T_nominal_value=owcjlhxdxh  Q_specify=off  Q_priority=None  Q=jawtmfuqev W  Q_nominal_specify=off  Q_nominal_unit=W  Q_nominal_value=amvswbkqpm
      settings: SourceProductName=Simscape Electrical  SourceProductBaseCode=PS  InternalSimscapePortConfiguration="{\"Bottom\":[],\"Left\":[{\"id\":\"A\",\"label\":\"A\",\"type\":\"foundation.thermal.thermal\"}],\"Right\":[{\"id\":\"B\",\"label\":\"B\",\"type\":\"foundation.thermal.thermal\"}],\"Top\":[]}"
  Redacted_4312 : PMIOPort  Side=Left
  Redacted_7440 : PMIOPort  Port=2  Side=Left
  Redacted_7574 : PMIOPort  Port=3  Side=Right
  Redacted_5998 : PMIOPort  Port=4  Side=Right
  Redacted_5346 : PMIOPort  Port=5  Side=Left
  Redacted_698 : PMIOPort  Port=6  Side=Right
  connections:
  Redacted_3861/LConn2 -- Redacted_7612/LConn1
  Redacted_6041/RConn1 -- Redacted_5346/RConn1
  Redacted_5998/RConn1 -- Redacted_5977/RConn2
  Redacted_1005/RConn1 -- Redacted_5977/RConn1 -- Redacted_698/RConn1
  Redacted_1354/RConn1 -- Redacted_6041/LConn1 -- Redacted_7612/RConn1
  Redacted_4312/RConn1 -- Redacted_3286/RConn1
  Redacted_3286/LConn1 -- Redacted_1005/LConn1
  Redacted_7574/RConn1 -- Redacted_1005/RConn2
  Redacted_3286/LConn2 -- Redacted_1354/LConn1
  Redacted_3861/RConn1 -- Redacted_5977/LConn1
  Redacted_3861/LConn1 -- Redacted_7440/RConn1

== system Electrical_System_2018b_obfs/Redacted_1221/Redacted_7996/Redacted_1/Redacted_4377/Redacted_6082/Redacted_1843 ==
  Neutral_Negative : Subsystem  VariantControl=Variant1
  Positive_Neutral : Subsystem  VariantControl=Variant3
  Redacted_8971 : Subsystem  VariantControl=Variant2
  Redacted_2601 : PMIOPort  Side=Left
  Redacted_5367 : PMIOPort  Port=2  Side=Left
  Redacted_1109 : PMIOPort  Port=3  Side=Left
  Redacted_4235 : PMIOPort  Port=4  Side=Right
  Redacted_9086 : PMIOPort  Port=5  Side=Right

== system Electrical_System_2018b_obfs/Redacted_1221/Redacted_7996/Redacted_1/Redacted_4377/Redacted_6082/Redacted_1901 ==
  Redacted_1229 : ee_lib/Passive/Thermal/Thermal Resistor  R=hfneeleggr K/W  T_specify=off  T_priority=None  T=dnmeqksrrm K  T_nominal_specify=off  T_nominal_unit=K  T_nominal_value=uhclxpopbh  Q_specify=off  Q_priority=None  Q=nyzppyukeu W  Q_nominal_specify=off  Q_nominal_unit=W  Q_nominal_value=mrympoiojz
      settings: SourceProductName=Simscape Electrical  SourceProductBaseCode=PS  InternalSimscapePortConfiguration="{\"Bottom\":[],\"Left\":[{\"id\":\"A\",\"label\":\"A\",\"type\":\"foundation.thermal.thermal\"}],\"Right\":[{\"id\":\"B\",\"label\":\"B\",\"type\":\"foundation.thermal.thermal\"}],\"Top\":[]}"
  Redacted_1317 : ee_lib/Passive/Thermal/Thermal Resistor  R=ddtrqjrhjn K/W  T_specify=off  T_priority=None  T=myvnfneauu K  T_nominal_specify=off  T_nominal_unit=K  T_nominal_value=vndthaumwj  Q_specify=off  Q_priority=None  Q=jvrrmptdue W  Q_nominal_specify=off  Q_nominal_unit=W  Q_nominal_value=zyzovxzrox
      settings: SourceProductName=Simscape Electrical  SourceProductBaseCode=PS  InternalSimscapePortConfiguration="{\"Bottom\":[],\"Left\":[{\"id\":\"A\",\"label\":\"A\",\"type\":\"foundation.thermal.thermal\"}],\"Right\":[{\"id\":\"B\",\"label\":\"B\",\"type\":\"foundation.thermal.thermal\"}],\"Top\":[]}"
  Redacted_2918 : ee_lib/Semiconductors & Converters/Diode  ModelType=tboxenabfk  Vf=ysocghjvnj V  Ron=igyyqbbazt Ohm  Goff=wrcmatehqh S  prmExp=umofwxphaz  I12=boewnunols A  V12=agfxygazzy V  IS=yxpwlphqya A  ec=ezskytlukg  I1=hfmdeevxjm A  V1=lbjfenfgli V  RS=crmaftxtdn Ohm  Tmeas=rzhxrfhrws degC  N_series=qhotvmyapg  N_parallel=dcamtsthwp  Rz=qwnnbscosu Ohm  BV=bgsuezylxr V  C_param=jefhggiqkq  CJ=nrftpgzbwn pF  CJ0=vpkmzxlujx pF  VJ=nqopqysaak V  Mgrad=jnpgifqefs  Vvec=cniqwxpvbi V  Cvec=plwpepcsqe pF  FC=gzewllqrkw  Q_param=xlnrldobms  iRM=ytqzliqbll A  iF=svsqnejsfr A  didt=lrnrbryckm A/us  trr_factor=qpcgqhjpel  trr=emvijkzjdz ns  Qrr=ykzfmghaqw s*uA  TT=cegrsucons ns  tau=hhbhhwwsxm ns  T_param=jxhekmoycn  IS_T2=cnunlqxwqa A  I1_T2=tqdiqvzzvb A  V1_T2=ukgedxicts V  Tmeas2=ypzgidmcky degC  EG_param=ahptxqtjkj  EG=pprjzflisz eV  XTI_param=luwukgfqqn  XTI=bnvhtyteod  dBVdT=loswkuonel V/K  Tdevice=ctewjlisga degC  i_specify=off  i_priority=None  i=kufuhybcxo A  i_nominal_specify=off  i_nominal_unit=A  i_nominal_value=fnodmzekrv  v_specify=off  v_priority=None  v=bvjjoninjh V  v_nominal_specify=off  v_nominal_unit=V  v_nominal_value=wmrqkzdvam  i_capacitor_specify=off  i_capacitor_priority=None  i_capacitor=sawezjxpgh A  i_capacitor_nominal_specify=off  i_capacitor_nominal_unit=A  i_capacitor_nominal_value=dzrakfqruq  v_capacitor_specify=off  v_capacitor_priority=None  v_capacitor=ckefveljbv V  v_capacitor_nominal_specify=off  v_capacitor_nominal_unit=V  v_capacitor_nominal_value=zlbmprnqfe  power_dissipated_specify=off  power_dissipated_priority=None  power_dissipated=npelzyxkbr W  power_dissipated_nominal_specify=off  power_dissipated_nominal_unit=W  power_dissipated_nominal_value=xyqqsiyxsx  thermal_network_parameterization=cmpqaimztb  Rth=fyfjdoegdn K/W  Rth_Foster=ouazsjqzqc K/W  thermal_mass_parameterization=uskugrezwe  thermal_mass=kfppvbxohl J/K  thermal_mass_Foster=iohubghcog J/K  thermal_time_constant=tbegstwujr s  thermal_time_constant_Foster=kbaqkpxwop s  thermal_mass_initial_temperatures=tmxmgoawom degC
      settings: SourceProductName=Simscape Electrical  InternalSimscapePortConfiguration="{\"Bottom\":[],\"Left\":[{\"id\":\"p\",\"label\":\"\",\"type\":\"foundation.electrical.electrical\"},{\"id\":\"H\",\"label\":\"H\",\"type\":\"foundation.thermal.thermal\"}],\"Right\":[{\"id\":\"n\",\"label\":\"\",\"type\":\"foundation.electrical.electrical\"}],\"Top\":[]}"
  Redacted_3887 : ee_lib/Semiconductors & Converters/Diode  ModelType=kgpqvwzuvf  Vf=pusmgjlfhw V  Ron=zdvhkofkio Ohm  Goff=rrsomwrhky S  prmExp=puvexjufpm  I12=tlbhkktqov A  V12=jgzzzcxugv V  IS=pqeeblyemi A  ec=yagdawcefa  I1=baiumjodsv A  V1=kvrziecayr V  RS=emddjdnqya Ohm  Tmeas=kukopsdiuw degC  N_series=rabuyhqlar  N_parallel=fzdlculjid  Rz=oyqbhoxixc Ohm  BV=powcerqowi V  C_param=aeoqkmsqgo  CJ=omumwwbzoq pF  CJ0=sznaxolwxw pF  VJ=kdgpnhjdki V  Mgrad=owoxwkiptx  Vvec=yphehuqnex V  Cvec=yioiudmgas pF  FC=diwfpfnlom  Q_param=cswgmtympe  iRM=nsikknuycn A  iF=udnoipznau A  didt=omhhheqqis A/us  trr_factor=kiajvubcqx  trr=eifapbzssj ns  Qrr=igpekaohrl s*uA  TT=jucdrpilud ns  tau=lahsbpxgyi ns  T_param=vnthpegzri  IS_T2=edtnoyclnw A  I1_T2=emvajrspsy A  V1_T2=nghezzebkw V  Tmeas2=etfqwqeleu degC  EG_param=fmhucqmugz  EG=ytvyyycxld eV  XTI_param=kxpyactpjk  XTI=ijcctumawz  dBVdT=mveoqdoxea V/K  Tdevice=rasndouawu degC  i_specify=off  i_priority=None  i=middmtxema A  i_nominal_specify=off  i_nominal_unit=A  i_nominal_value=ulcnzrhotg  v_specify=off  v_priority=None  v=cirgoxespi V  v_nominal_specify=off  v_nominal_unit=V  v_nominal_value=dnkswukuqy  i_capacitor_specify=off  i_capacitor_priority=None  i_capacitor=uvmqwudjqx A  i_capacitor_nominal_specify=off  i_capacitor_nominal_unit=A  i_capacitor_nominal_value=tjhsaljlzi  v_capacitor_specify=off  v_capacitor_priority=None  v_capacitor=gtauwsvkmg V  v_capacitor_nominal_specify=off  v_capacitor_nominal_unit=V  v_capacitor_nominal_value=yrtxkgmrjc  power_dissipated_specify=off  power_dissipated_priority=None  power_dissipated=gejrmthogs W  power_dissipated_nominal_specify=off  power_dissipated_nominal_unit=W  power_dissipated_nominal_value=fnkdipvfax  thermal_network_parameterization=brstcitzoq  Rth=qauyoickxf K/W  Rth_Foster=pcmfvqnjph K/W  thermal_mass_parameterization=csstahwskj  thermal_mass=uinbpeizom J/K  thermal_mass_Foster=udgsofajzw J/K  thermal_time_constant=fbszgisaxv s  thermal_time_constant_Foster=qzpyvzuxkn s  thermal_mass_initial_temperatures=tcrrrnbkcb degC
      settings: SourceProductName=Simscape Electrical  InternalSimscapePortConfiguration="{\"Bottom\":[],\"Left\":[{\"id\":\"p\",\"label\":\"\",\"type\":\"foundation.electrical.electrical\"},{\"id\":\"H\",\"label\":\"H\",\"type\":\"foundation.thermal.thermal\"}],\"Right\":[{\"id\":\"n\",\"label\":\"\",\"type\":\"foundation.electrical.electrical\"}],\"Top\":[]}"
  Redacted_5062 : fl_lib/Electrical/Electrical Elements/Switch  R_closed=ajgjjzldor Ohm  G_open=aanuvbeift 1/Ohm  Threshold=fyvpcwnmem  i_specify=off  i_priority=None  i=farnwkyrka A  i_nominal_specify=off  i_nominal_unit=A  i_nominal_value=uzlteuglkb  v_specify=off  v_priority=None  v=tekycmpguo V  v_nominal_specify=off  v_nominal_unit=V  v_nominal_value=hyrhbabztl
      settings: SourceProductName=Simscape
  Redacted_6145 : fl_lib/Electrical/Electrical Elements/Switch  R_closed=wzxtffzhqk Ohm  G_open=ttmifnbefi 1/Ohm  Threshold=zzdsjwvyov  i_specify=off  i_priority=None  i=wibaukydmt A  i_nominal_specify=off  i_nominal_unit=A  i_nominal_value=shaiddzzkm  v_specify=off  v_priority=None  v=adhjlkibew V  v_nominal_specify=off  v_nominal_unit=V  v_nominal_value=ctlxurrbzu
      settings: SourceProductName=Simscape
  Redacted_8303 : ee_lib/Passive/Thermal/Thermal Resistor  R=dcadmadufn K/W  T_specify=off  T_priority=None  T=kapvbwdbts K  T_nominal_specify=off  T_nominal_unit=K  T_nominal_value=ghgowxtkgp  Q_specify=off  Q_priority=None  Q=amzvaiirbc W  Q_nominal_specify=off  Q_nominal_unit=W  Q_nominal_value=ptxjogujxs
      settings: SourceProductName=Simscape Electrical  SourceProductBaseCode=PS  InternalSimscapePortConfiguration="{\"Bottom\":[],\"Left\":[{\"id\":\"A\",\"label\":\"A\",\"type\":\"foundation.thermal.thermal\"}],\"Right\":[{\"id\":\"B\",\"label\":\"B\",\"type\":\"foundation.thermal.thermal\"}],\"Top\":[]}"
  Redacted_8116 : PMIOPort  Side=Left
  Redacted_9290 : PMIOPort  Port=2  Side=Left
  Redacted_6411 : PMIOPort  Port=3  Side=Right
  Redacted_9481 : PMIOPort  Port=4  Side=Right
  Redacted_1243 : PMIOPort  Port=5  Side=Left
  Redacted_5181 : PMIOPort  Port=6  Side=Right
  connections:
  Redacted_3887/LConn1 -- Redacted_9290/RConn1
  Redacted_3887/RConn1 -- Redacted_6145/LConn1
  Redacted_2918/LConn2 -- Redacted_1229/LConn1
  Redacted_6411/RConn1 -- Redacted_5062/RConn2
  Redacted_2918/LConn1 -- Redacted_5062/LConn1
  Redacted_8116/RConn1 -- Redacted_2918/RConn1
  Redacted_1317/RConn1 -- Redacted_8303/LConn1 -- Redacted_1229/RConn1
  Redacted_5181/RConn1 -- Redacted_6145/RConn1 -- Redacted_5062/RConn1
  Redacted_9481/RConn1 -- Redacted_6145/RConn2
  Redacted_8303/RConn1 -- Redacted_1243/RConn1
  Redacted_3887/LConn2 -- Redacted_1317/LConn1

== system Electrical_System_2018b_obfs/Redacted_1221/Redacted_7996/Redacted_1/Redacted_4377/Redacted_6082/Redacted_2005 ==
  Neutral_Negative : Subsystem  VariantControl=Variant1
  Positive_Neutral : Subsystem  VariantControl=Variant3
  Redacted_335 : Subsystem  VariantControl=Variant2
  Redacted_8266 : PMIOPort  Side=Left
  Redacted_1423 : PMIOPort  Port=2  Side=Left
  Redacted_7633 : PMIOPort  Port=3  Side=Left
  Redacted_8552 : PMIOPort  Port=4  Side=Right
  Redacted_2441 : PMIOPort  Port=5  Side=Right

== system Electrical_System_2018b_obfs/Redacted_1221/Redacted_7996/Redacted_1/Redacted_4377/Redacted_6082/Redacted_2122 ==
  Neutral_Negative : Subsystem  VariantControl=Variant1
  Positive_Neutral : Subsystem  VariantControl=Variant3
  Redacted_1391 : Subsystem  VariantControl=Variant2
  Redacted_659 : PMIOPort  Side=Left
  Redacted_1619 : PMIOPort  Port=2  Side=Left
  Redacted_5171 : PMIOPort  Port=3  Side=Left
  Redacted_2219 : PMIOPort  Port=4  Side=Right
  Redacted_5591 : PMIOPort  Port=5  Side=Right
